simulink model "MSFartoystyring_compensated"  (R2019a)
settings: Solver=ode45  StartTime=tstart  StopTime=tstop  RelTol=1e-3  EnableMultiTasking=on
values from neighbouring files (symbols this model uses):
  c = 1    [compensated.m]
  p0 = [1000, 700]    [compensated.m]
  psi0 = deg2rad(60)    [compensated.m]
  r0 = 0    [compensated.m]
  tsamp = 10    [compensated.m]
  v0 = [6.63 0]'    [compensated.m]
undefined symbols (not defined in the file or in its folder): chi2psi, delta_max, distance_threshold, heading_controller, K_iu, K_psi, K_pu, L_pp, msfartoystyring, n_max, numeric_threshold, speed_controller, T_psi, U2u, WP
settings Model: ExtModeAutoUpdateStatusClock=off  Creator=christh  LastModifiedBy=martiege
settings DataIOCC: LimitDataPoints=on  SaveFormat=Array  SignalLoggingSaveFormat=ModelDataLogs  ReturnWorkspaceOutputs=off
settings OptimizationCC: ExpressionDepthLimit=2147483647  InitFltsAndDblsToZero=on  LifeSpan=inf
settings DebuggingCC: UnderspecifiedInitializationDetection=Classic  MergeDetectMultiDrivingBlocksExec=none  SolverPrmCheckMsg=warning  FcnCallInpInsideContextMsg=warning  StateNameClashWarn=warning  SFUnexpectedBacktrackingDiag=warning  SFNoUnconditionalDefaultTransitionDiag=warning  ArithmeticOperatorsInVariantConditions=warning
settings HardwareCC: ProdBitPerPointer=32  ProdBitPerSizeT=32  ProdBitPerPtrDiffT=32  ProdLargestAtomicFloat=None  ProdIntDivRoundTo=Undefined  ProdEndianess=Unspecified  ProdWordSize=32  ProdHWDeviceType=32-bit Generic
settings ModelReferenceCC: PropagateSignalLabelsOutOfModel=off
settings SFSimCC: SimUseLocalCustomCode=off
settings RTWCC: RTWUseLocalCustomCode=off
settings CodeAppCC: StateflowObjectComments=on
settings GRTTargetCC: TargetLangStandard=C89/C90 (ANSI)  GeneratePreprocessorConditionals=Disable all  CombineOutputUpdateFcns=off  GRTInterface=on
settings ConfigComp: CovMetricSettings=dw  CovHtmlReporting=on  CovSaveCumulativeToWorkspaceVar=on  CovSaveSingleToWorkspaceVar=on  CovExternalEMLEnable=off

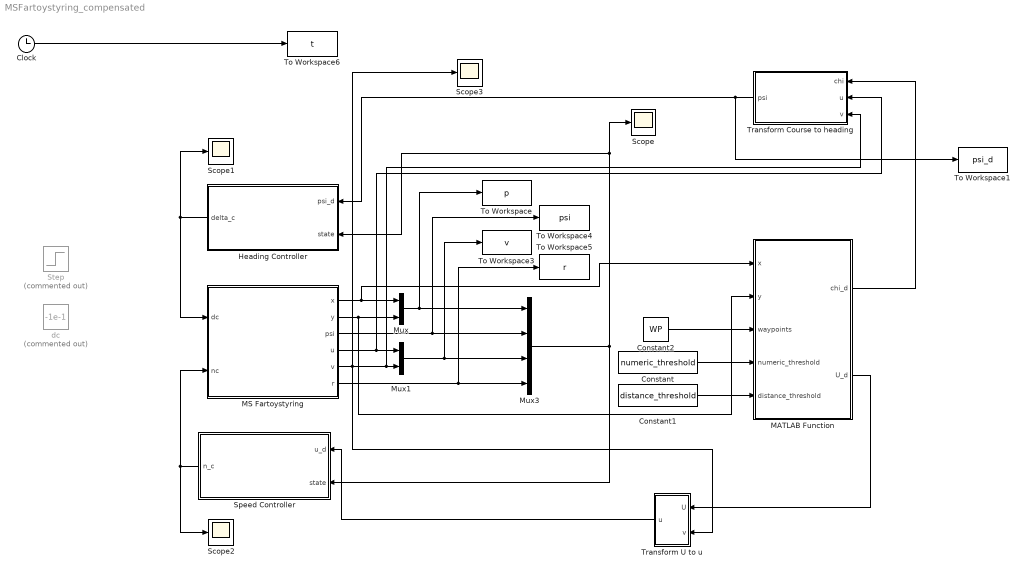
== system MSFartoystyring_compensated ==
  Clock : Clock
  Constant : Constant  Value=numeric_threshold
  Constant1 : Constant  Value=distance_threshold
  Constant2 : Constant  Value=WP
  "Heading Controller " : Subsystem
  MATLAB Function : MATLAB Function  TreatAsAtomicUnit=on
  MS Fartoystyring : Subsystem  mask(MS Fartoystyring for Assignment 3 G&C){x0=p0(1), y0=p0(2), u0=v0(1), v0=v0(2), psi0=psi0, r0=r0, c=c}
      mask prompts: x0 "x(t0) (m)"; y0 "y(t0) (m)"; u0 "u(t0) (m/s)"; v0 "v(t0) (m/s)"; psi0 "psi(t0) (rad)"; r0 "r(t0) (rad/s)"; c "current (0 or 1)"
      mask help:
      | Block corresponding to Figure 1 in the assignment text. Gives the response of the ship.
      |
      | The design speed of MS Fartoystyring is u=8.23 m/s.
      |
      | Input:
      | dc: commanded rudder (rad), dmax=25*pi/180
      | nc: commanded shaft speed (rad/s), nmax=85*2*pi/60
      |
      | Output:
      | x: north pos (m)
      | y: east pos (m)
      | u: surge (m/s)
      | v: sway (m/s)
      | psi: heading (rad)
      | r: yaw (rad/s)
      mask Help: Comments, bugs and help requests can be directed to the TA. Email on course website.
  Mux : Mux  Inputs=2
  Mux1 : Mux  Inputs=2
  Mux3 : Mux
  Scope{,1..3} (4 alike) : Scope
  Speed Controller : Subsystem
  Step : Step  Commented=on  Time=0  After=-deg2rad(25)  SampleTime=0
  To Workspace : ToWorkspace  VariableName=p  SampleTime=tsamp
  To Workspace1 : ToWorkspace  VariableName=psi_d  SampleTime=tsamp
  To Workspace3 : ToWorkspace  VariableName=v  SampleTime=tsamp
  To Workspace4 : ToWorkspace  VariableName=psi  SampleTime=tsamp
  To Workspace5 : ToWorkspace  VariableName=r  SampleTime=tsamp
  To Workspace6 : ToWorkspace  VariableName=t  SampleTime=tsamp
  Transform Course to heading : Subsystem
  Transform U to u : Subsystem
  dc : Constant  Commented=on  Value=-1e-1
  wires:
  Clock/1 -> To Workspace6/1
  MS Fartoystyring/1(x) -> MATLAB Function/1(x), Mux/1
  MS Fartoystyring/2(y) -> MATLAB Function/2(y), Mux/2
  MS Fartoystyring/4(u) -> Transform Course to heading/2(u), Mux1/1
  MS Fartoystyring/5(v) -> Transform U to u/2(v), Scope3/1, Transform Course to heading/3(v), Mux1/2
  Mux/1 -> To Workspace/1, Mux3/1
  Mux1/1 -> To Workspace3/1, Mux3/3
  MS Fartoystyring/3(psi) -> To Workspace4/1, Mux3/2
  MS Fartoystyring/6(r) -> To Workspace5/1, Mux3/4
  Mux3/1 -> "Heading Controller "/2(state), Scope/1, Speed Controller/2(state)
  "Heading Controller "/1(delta_c) -> Scope1/1, MS Fartoystyring/1(dc)
  Speed Controller/1(n_c) -> MS Fartoystyring/2(nc), Scope2/1
  Constant2/1 -> MATLAB Function/3(waypoints)
  Constant/1 -> MATLAB Function/4(numeric_threshold)
  Constant1/1 -> MATLAB Function/5(distance_threshold)
  MATLAB Function/1(chi_d) -> Transform Course to heading/1(chi)
  Transform Course to heading/1(psi) -> "Heading Controller "/1(psi_d), To Workspace1/1
  MATLAB Function/2(U_d) -> Transform U to u/1(U)
  Transform U to u/1(u) -> Speed Controller/1(u_d)

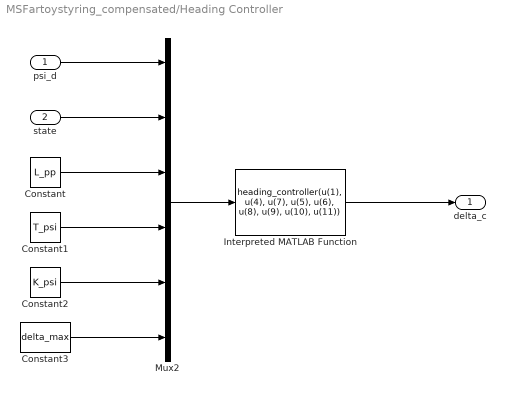
== system MSFartoystyring_compensated/Heading Controller  ==
  psi_d : Inport
  state : Inport  Port=2
  Constant : Constant  Value=L_pp
  Constant1 : Constant  Value=T_psi
  Constant2 : Constant  Value=K_psi
  Constant3 : Constant  Value=delta_max
  Interpreted MATLAB Function : MATLABFcn  MATLABFcn=heading_controller(u(1), u(4), u(7), u(5), u(6), u(8), u(9), u(10), u(11))
  Mux2 : Mux  Inputs=6
  delta_c : Outport
  wires:
  Constant3/1 -> Mux2/6
  Constant/1 -> Mux2/3
  psi_d/1 -> Mux2/1
  Constant1/1 -> Mux2/4
  state/1 -> Mux2/2
  Interpreted MATLAB Function/1 -> delta_c/1
  Mux2/1 -> Interpreted MATLAB Function/1
  Constant2/1 -> Mux2/5

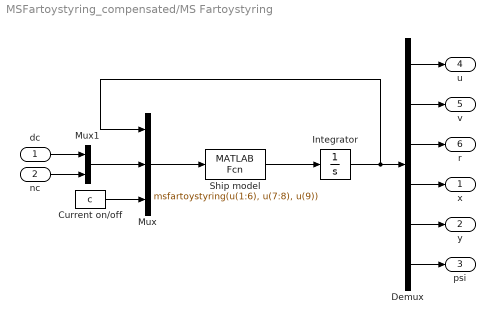
== system MSFartoystyring_compensated/MS Fartoystyring ==
  dc : Inport
  nc : Inport  Port=2
  Current on/off : Constant  Value=c
  Demux : Demux  Outputs=6
  Integrator : Integrator  InitialCondition=[u0 v0 r0 x0 y0 psi0]'
  Mux : Mux  Inputs=3
  Mux1 : Mux  Inputs=2
  Ship model : MATLABFcn  MATLABFcn=msfartoystyring(u(1:6), u(7:8), u(9))  OutputDimensions=6
  x : Outport
  y : Outport  Port=2
  psi : Outport  Port=3
  u : Outport  Port=4
  v : Outport  Port=5
  r : Outport  Port=6
  wires:
  Integrator/1 -> Mux/1, Demux/1
  Mux1/1 -> Mux/2
  dc/1 -> Mux1/1
  nc/1 -> Mux1/2
  Demux/1 -> u/1
  Demux/2 -> v/1
  Demux/3 -> r/1
  Demux/4 -> x/1
  Demux/5 -> y/1
  Demux/6 -> psi/1
  Current on/off/1 -> Mux/3
  Ship model/1 -> Integrator/1
  Mux/1 -> Ship model/1

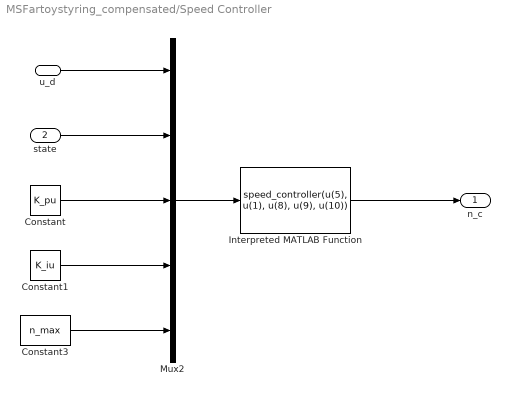
== system MSFartoystyring_compensated/Speed Controller ==
  u_d : Inport
  state : Inport  Port=2
  Constant : Constant  Value=K_pu
  Constant1 : Constant  Value=K_iu
  Constant3 : Constant  Value=n_max
  Interpreted MATLAB Function : MATLABFcn  MATLABFcn=speed_controller(u(5), u(1), u(8), u(9), u(10))
  Mux2 : Mux  Inputs=5
  n_c : Outport
  wires:
  Interpreted MATLAB Function/1 -> n_c/1
  Mux2/1 -> Interpreted MATLAB Function/1
  u_d/1 -> Mux2/1
  state/1 -> Mux2/2
  Constant/1 -> Mux2/3
  Constant1/1 -> Mux2/4
  Constant3/1 -> Mux2/5

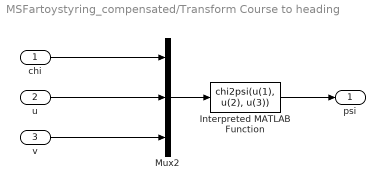
== system MSFartoystyring_compensated/Transform Course to heading ==
  chi : Inport
  u : Inport  Port=2
  v : Inport  Port=3
  Interpreted MATLAB Function : MATLABFcn  MATLABFcn=chi2psi(u(1), u(2), u(3))
  Mux2 : Mux  Inputs=3
  psi : Outport
  wires:
  u/1 -> Mux2/2
  Mux2/1 -> Interpreted MATLAB Function/1
  v/1 -> Mux2/3
  Interpreted MATLAB Function/1 -> psi/1
  chi/1 -> Mux2/1

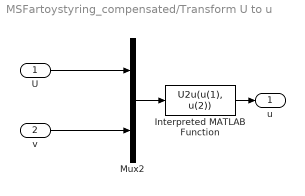
== system MSFartoystyring_compensated/Transform U to u ==
  U : Inport
  v : Inport  Port=2
  Interpreted MATLAB Function : MATLABFcn  MATLABFcn=U2u(u(1), u(2))
  Mux2 : Mux  Inputs=2
  u : Outport
  wires:
  Mux2/1 -> Interpreted MATLAB Function/1
  U/1 -> Mux2/1
  Interpreted MATLAB Function/1 -> u/1
  v/1 -> Mux2/2

== matlab function MSFartoystyring_compensated/MATLAB Function ==
  settings: updateMethod=DISCRETE
  data: chi_d output; x input; U_d output; y input; waypoints input; numeric_threshold input; distance_threshold input
function [chi_d, U_d] = fcn(x, y, waypoints, ...
    numeric_threshold, distance_threshold)

[U_d, chi_d] = guidance(x, y, waypoints, ...
    numeric_threshold, distance_threshold);
